simulink model "AR4FullPositionControl"  (R2026a)
settings: Solver=FixedStepAuto  StopTime=inf  FixedStep=3e-5
PreLoadFcn:
  | load('last_pos.mat');
StopFcn:
  | save('last_pos.mat', 'posJ6', 'posJ5', 'posJ4', 'posJ3', 'posJ2', 'posJ1', 'lastX', 'lastY', 'lastZ');
undefined symbols (not defined in the file): targetColor, targetGo, targetX, targetY, targetZ
libraries: arduinolib x31
(part 1 of 3)
settings Model: SILPILModeSetting=veronly  ExtModeTrigDuration=2  TunableVars=px  TunableVarsStorageClass=ExportedGlobal  Creator=abdnuris  LastModifiedBy=abdnuris
settings HardwareCC: ProdLargestAtomicInteger=Long  ProdLargestAtomicFloat=Double  ProdHWDeviceType=ARM Compatible->ARM Cortex
settings RTWCC: SystemTargetFile=ert.tlc  HardwareBoard=Teensy 4.1 (Arduino Compatible)  TLCOptions=-aInlineSetEventsForThisBaseRateFcn=TLC_FALSE -aSuppressMultiTaskScheduler=TLC_FALSE -aRateBasedStepFcn=1  Toolchain=Arduino ARM M7  Description=Embedded Coder
settings ERTTargetCC: ExtModeTransport=3.0  ExtModeAutomaticAllocSize=off  ExtModeStaticAllocSize=65536.0  SupportContinuousTime=on  SupportVariableSizeSignals=on

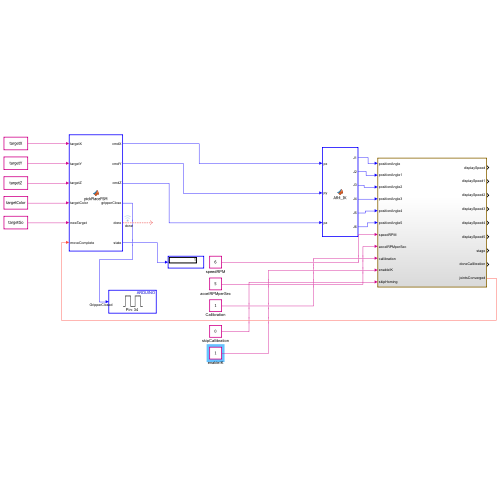
[thumbnail: Simulink's stored preview of the top-level diagram]
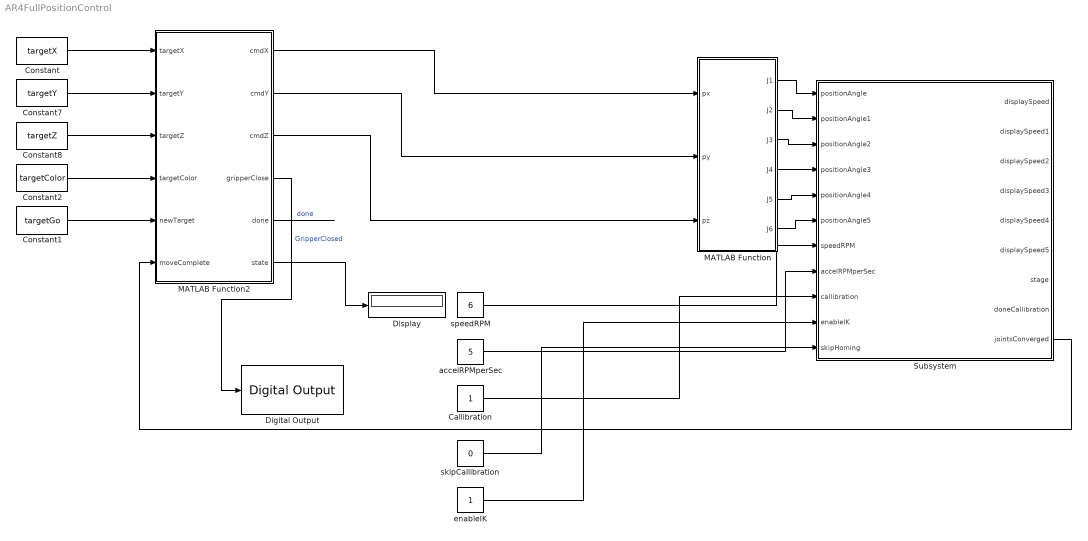
== system AR4FullPositionControl ==
  Callibration : Constant
  Constant : Constant  Value=targetX
  Constant1 : Constant  Value=targetGo
  Constant2 : Constant  Value=targetColor
  Constant7 : Constant  Value=targetY
  Constant8 : Constant  Value=targetZ
  Digital Output : arduinolib/Digital Output  pinNumber=34  Direction=output  blockPlatform=arduino
  Display : Display
  MATLAB Function : MATLAB Function  TreatAsAtomicUnit=on  SystemSampleTime=0.0075
  MATLAB Function2 : MATLAB Function  TreatAsAtomicUnit=on  SystemSampleTime=0.03
  Subsystem : Subsystem
  accelRPMperSec : Constant  Value=5
  enableIK : Constant
  skipCallibration : Constant  Value=0
  speedRPM : Constant  Value=6
  wires:
  MATLAB Function/2(J2) -> Subsystem/2(positionAngle1)
  MATLAB Function/3(J3) -> Subsystem/3(positionAngle2)
  MATLAB Function/4(J4) -> Subsystem/4(positionAngle3)
  MATLAB Function/5(J5) -> Subsystem/5(positionAngle4)
  MATLAB Function/6(J6) -> Subsystem/6(positionAngle5)
  MATLAB Function/1(J1) -> Subsystem/1(positionAngle)
  speedRPM/1 -> Subsystem/7(speedRPM)
  accelRPMperSec/1 -> Subsystem/8(accelRPMperSec)
  Callibration/1 -> Subsystem/9(callibration)
  enableIK/1 -> Subsystem/10(enableIK)
  MATLAB Function2/4(gripperClose) -> Digital Output/1  "GripperClosed"
  skipCallibration/1 -> Subsystem/11(skipHoming)
  Constant7/1 -> MATLAB Function2/2(targetY)
  Constant/1 -> MATLAB Function2/1(targetX)
  Constant8/1 -> MATLAB Function2/3(targetZ)
  Constant1/1 -> MATLAB Function2/5(newTarget)
  MATLAB Function2/5(done) -> ?  "done"
  Subsystem/9(jointsConverged) -> MATLAB Function2/6(moveComplete)
  MATLAB Function2/6(state) -> Display/1
  MATLAB Function2/1(cmdX) -> MATLAB Function/1(px)
  MATLAB Function2/3(cmdZ) -> MATLAB Function/3(pz)
  MATLAB Function2/2(cmdY) -> MATLAB Function/2(py)
  Constant2/1 -> MATLAB Function2/4(targetColor)

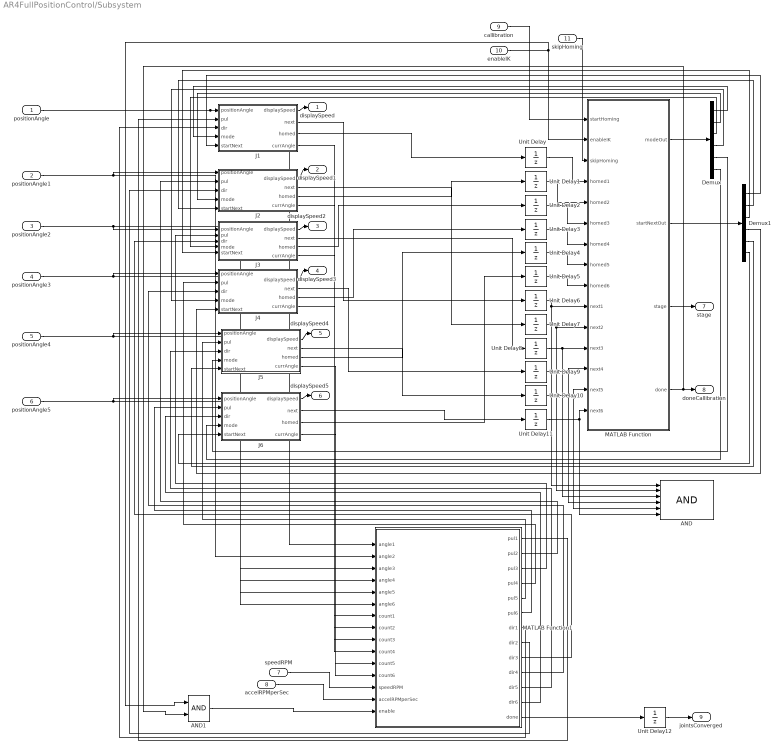
== system AR4FullPositionControl/Subsystem ==
  positionAngle : Inport
  positionAngle1 : Inport  Port=2
  positionAngle2 : Inport  Port=3
  positionAngle3 : Inport  Port=4
  positionAngle4 : Inport  Port=5
  positionAngle5 : Inport  Port=6
  speedRPM : Inport  Port=7
  accelRPMperSec : Inport  Port=8
  callibration : Inport  Port=9
  enableIK : Inport  Port=10
  skipHoming : Inport  Port=11
  AND : Logic  Inputs=6  IconShape=distinctive  AllPortsSameDT=off  OutDataTypeStr=boolean
  AND1 : Logic  IconShape=distinctive  AllPortsSameDT=off  OutDataTypeStr=boolean
  Demux : Demux  Outputs=6
  Demux1 : Demux  Outputs=6
  J1 : Subsystem
  J2 : Subsystem
  J3 : Subsystem
  J4 : Subsystem
  J5 : Subsystem
  J6 : Subsystem
  MATLAB Function : MATLAB Function  TreatAsAtomicUnit=on  SystemSampleTime=0.0075
  MATLAB Function1 : MATLAB Function  TreatAsAtomicUnit=on  SystemSampleTime=3e-5
  Unit Delay{,1..11} (12 alike) : UnitDelay  SampleTime=-1
  Unit Delay12 : UnitDelay  InitialCondition=false  SampleTime=-1
  displaySpeed : Outport
  displaySpeed1 : Outport  Port=2
  displaySpeed2 : Outport  Port=3
  displaySpeed3 : Outport  Port=4
  displaySpeed4 : Outport  Port=5
  displaySpeed5 : Outport  Port=6
  stage : Outport  Port=7
  doneCallibration : Outport  Port=8
  jointsConverged : Outport  Port=9
  wires:
  positionAngle4/1 -> MATLAB Function1/5(angle5), J5/1(positionAngle)
  MATLAB Function1/6(pul6) -> J6/2(pul)
  J2/2(next) -> Unit Delay7/1
  J6/1(displaySpeed) -> displaySpeed5/1
  positionAngle5/1 -> MATLAB Function1/6(angle6), J6/1(positionAngle)
  J3/2(next) -> Unit Delay8/1
  positionAngle2/1 -> MATLAB Function1/3(angle3), J3/1(positionAngle)
  J4/2(next) -> Unit Delay9/1
  positionAngle1/1 -> MATLAB Function1/2(angle2), J2/1(positionAngle)
  positionAngle/1 -> MATLAB Function1/1(angle1), J1/1(positionAngle)
  positionAngle3/1 -> MATLAB Function1/4(angle4), J4/1(positionAngle)
  J2/1(displaySpeed) -> displaySpeed1/1
  J4/1(displaySpeed) -> displaySpeed3/1
  J5/1(displaySpeed) -> displaySpeed4/1
  J3/1(displaySpeed) -> displaySpeed2/1
  J5/2(next) -> Unit Delay10/1
  J1/1(displaySpeed) -> displaySpeed/1
  J6/2(next) -> Unit Delay11/1
  MATLAB Function1/12(dir6) -> J6/3(dir)
  J1/3(homed) -> Unit Delay/1
  J2/3(homed) -> Unit Delay1/1
  J3/3(homed) -> Unit Delay2/1
  J4/3(homed) -> Unit Delay3/1
  J5/3(homed) -> Unit Delay4/1
  J6/3(homed) -> Unit Delay5/1
  callibration/1 -> MATLAB Function/1(startHoming)
  MATLAB Function/1(modeOut) -> Demux/1
  Demux/1 -> J1/4(mode)
  Demux/2 -> J2/4(mode)
  Demux/3 -> J3/4(mode)
  Demux/4 -> J4/4(mode)
  Demux/5 -> J5/4(mode)
  Demux/6 -> J6/4(mode)
  MATLAB Function/2(startNextOut) -> Demux1/1
  Demux1/1 -> J1/5(startNext)
  Demux1/2 -> J2/5(startNext)
  Demux1/3 -> J3/5(startNext)
  Demux1/4 -> J4/5(startNext)
  Demux1/5 -> J5/5(startNext)
  Demux1/6 -> J6/5(startNext)
  enableIK/1 -> MATLAB Function/2(enableIK), AND1/1
  MATLAB Function/3(stage) -> stage/1
  MATLAB Function/4(done) -> AND1/2, doneCallibration/1
  Unit Delay/1 -> MATLAB Function/4(homed1)
  Unit Delay1/1 -> MATLAB Function/5(homed2)
  Unit Delay2/1 -> MATLAB Function/6(homed3)
  Unit Delay3/1 -> MATLAB Function/7(homed4)
  Unit Delay4/1 -> MATLAB Function/8(homed5)
  Unit Delay5/1 -> MATLAB Function/9(homed6)
  Unit Delay6/1 -> AND/1, MATLAB Function/10(next1)
  Unit Delay7/1 -> AND/2, MATLAB Function/11(next2)
  Unit Delay8/1 -> AND/3, MATLAB Function/12(next3)
  Unit Delay9/1 -> AND/4, MATLAB Function/13(next4)
  Unit Delay10/1 -> AND/5, MATLAB Function/14(next5)
  Unit Delay11/1 -> AND/6, MATLAB Function/15(next6)
  J1/2(next) -> Unit Delay6/1
  J1/4(currAngle) -> MATLAB Function1/7(count1)
  J2/4(currAngle) -> MATLAB Function1/8(count2)
  J3/4(currAngle) -> MATLAB Function1/9(count3)
  J4/4(currAngle) -> MATLAB Function1/10(count4)
  J5/4(currAngle) -> MATLAB Function1/11(count5)
  J6/4(currAngle) -> MATLAB Function1/12(count6)
  speedRPM/1 -> MATLAB Function1/13(speedRPM)
  accelRPMperSec/1 -> MATLAB Function1/14(accelRPMperSec)
  MATLAB Function1/1(pul1) -> J1/2(pul)
  MATLAB Function1/2(pul2) -> J2/2(pul)
  MATLAB Function1/3(pul3) -> J3/2(pul)
  MATLAB Function1/4(pul4) -> J4/2(pul)
  MATLAB Function1/5(pul5) -> J5/2(pul)
  MATLAB Function1/10(dir4) -> J4/3(dir)
  MATLAB Function1/8(dir2) -> J2/3(dir)
  MATLAB Function1/7(dir1) -> J1/3(dir)
  MATLAB Function1/11(dir5) -> J5/3(dir)
  MATLAB Function1/9(dir3) -> J3/3(dir)
  skipHoming/1 -> MATLAB Function/3(skipHoming)
  Unit Delay12/1 -> jointsConverged/1
  MATLAB Function1/13(done) -> Unit Delay12/1
  AND1/1 -> MATLAB Function1/15(enable)

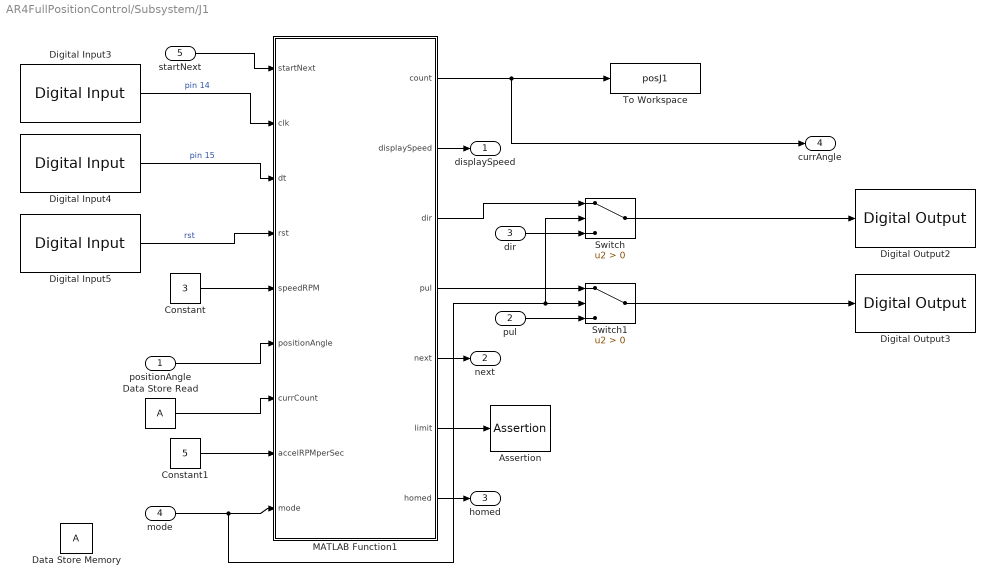
== system AR4FullPositionControl/Subsystem/J1 ==
  positionAngle : Inport
  pul : Inport  Port=2
  dir : Inport  Port=3
  mode : Inport  Port=4
  startNext : Inport  Port=5
  Assertion : Assertion  AssertionFailFcn="error(\"Limit J1\")"
  Constant : Constant  Value=3
  Constant1 : Constant  Value=5
  Data Store Memory : DataStoreMemory  WriteAfterWriteMsg=warning  InitialValue=posJ1  ShowAdditionalParam=off
  Data Store Read : DataStoreRead  IndexOptions=Index vector (dialog)  Indices=1  OutputSizes=1
  Digital Input3 : arduinolib/Digital Input  pinNumber=14  mode=Default  Direction=input  SampleTime=-1  blockPlatform=arduino
  Digital Input4 : arduinolib/Digital Input  pinNumber=15  mode=Default  Direction=input  SampleTime=-1  blockPlatform=arduino
  Digital Input5 : arduinolib/Digital Input  pinNumber=26  mode=Default  Direction=input  SampleTime=0.0015  blockPlatform=arduino
  Digital Output2 : arduinolib/Digital Output  pinNumber=1  Direction=output  blockPlatform=arduino
  Digital Output3 : arduinolib/Digital Output  pinNumber=0  Direction=output  blockPlatform=arduino
  MATLAB Function1 : MATLAB Function  TreatAsAtomicUnit=on  SystemSampleTime=3e-5
  Switch : Switch  Criteria=u2 > Threshold  SaturateOnIntegerOverflow=off  InputSameDT=off
  Switch1 : Switch  Criteria=u2 > Threshold  SaturateOnIntegerOverflow=off  InputSameDT=off
  To Workspace : ToWorkspace  VariableName=posJ1  SampleTime=0.0075
      settings: MaxDataPoints=1  Decimation=2
  displaySpeed : Outport
  next : Outport  Port=2
  homed : Outport  Port=3
  currAngle : Outport  Port=4
  wires:
  MATLAB Function1/6(limit) -> Assertion/1
  Digital Input4/1 -> MATLAB Function1/3(dt)  "pin 15"
  Data Store Read/1 -> MATLAB Function1/7(currCount)
  startNext/1 -> MATLAB Function1/1(startNext)
  Digital Input3/1 -> MATLAB Function1/2(clk)  "pin 14"
  Digital Input5/1 -> MATLAB Function1/4(rst)  "rst"
  positionAngle/1 -> MATLAB Function1/6(positionAngle)
  MATLAB Function1/2(displaySpeed) -> displaySpeed/1
  MATLAB Function1/5(next) -> next/1
  MATLAB Function1/7(homed) -> homed/1
  MATLAB Function1/1(count) -> currAngle/1, To Workspace/1
  Switch1/1 -> Digital Output3/1
  MATLAB Function1/3(dir) -> Switch/1
  mode/1 -> Switch1/2, Switch/2, MATLAB Function1/9(mode)
  MATLAB Function1/4(pul) -> Switch1/1
  dir/1 -> Switch/3
  pul/1 -> Switch1/3
  Switch/1 -> Digital Output2/1
  Constant/1 -> MATLAB Function1/5(speedRPM)
  Constant1/1 -> MATLAB Function1/8(accelRPMperSec)

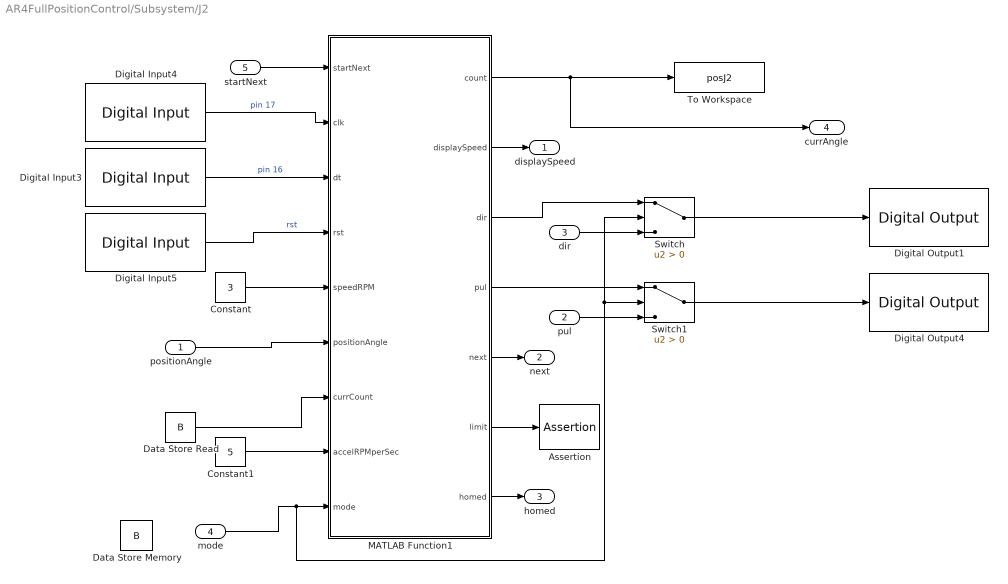
== system AR4FullPositionControl/Subsystem/J2 ==
  positionAngle : Inport
  pul : Inport  Port=2
  dir : Inport  Port=3
  mode : Inport  Port=4
  startNext : Inport  Port=5
  Assertion : Assertion  AssertionFailFcn="error(\"Limit J2\")"
  Constant : Constant  Value=3
  Constant1 : Constant  Value=5
  Data Store Memory : DataStoreMemory  DataStoreName=B  WriteAfterWriteMsg=warning  InitialValue=posJ2  ShowAdditionalParam=off
  Data Store Read : DataStoreRead  DataStoreName=B  IndexOptions=Index vector (dialog)  Indices=1  OutputSizes=1
  Digital Input3 : arduinolib/Digital Input  pinNumber=16  mode=Default  Direction=input  SampleTime=-1  blockPlatform=arduino
  Digital Input4 : arduinolib/Digital Input  pinNumber=17  mode=Default  Direction=input  SampleTime=-1  blockPlatform=arduino
  Digital Input5 : arduinolib/Digital Input  pinNumber=27  mode=Default  Direction=input  SampleTime=0.0015  blockPlatform=arduino
  Digital Output1 : arduinolib/Digital Output  pinNumber=3  Direction=output  blockPlatform=arduino
  Digital Output4 : arduinolib/Digital Output  pinNumber=2  Direction=output  blockPlatform=arduino
  MATLAB Function1 : MATLAB Function  TreatAsAtomicUnit=on
  Switch : Switch  Criteria=u2 > Threshold  SaturateOnIntegerOverflow=off  InputSameDT=off
  Switch1 : Switch  Criteria=u2 > Threshold  SaturateOnIntegerOverflow=off  InputSameDT=off
  To Workspace : ToWorkspace  VariableName=posJ2  SampleTime=0.0075
      settings: MaxDataPoints=1  Decimation=2
  displaySpeed : Outport
  next : Outport  Port=2
  homed : Outport  Port=3
  currAngle : Outport  Port=4
  wires:
  Digital Input4/1 -> MATLAB Function1/2(clk)  "pin 17"
  Digital Input5/1 -> MATLAB Function1/4(rst)  "rst"
  Digital Input3/1 -> MATLAB Function1/3(dt)  "pin 16"
  Data Store Read/1 -> MATLAB Function1/7(currCount)
  MATLAB Function1/6(limit) -> Assertion/1
  MATLAB Function1/5(next) -> next/1
  MATLAB Function1/2(displaySpeed) -> displaySpeed/1
  positionAngle/1 -> MATLAB Function1/6(positionAngle)
  MATLAB Function1/7(homed) -> homed/1
  startNext/1 -> MATLAB Function1/1(startNext)
  MATLAB Function1/1(count) -> currAngle/1, To Workspace/1
  MATLAB Function1/4(pul) -> Switch1/1
  MATLAB Function1/3(dir) -> Switch/1
  Switch1/1 -> Digital Output4/1
  Switch/1 -> Digital Output1/1
  mode/1 -> Switch/2, Switch1/2, MATLAB Function1/9(mode)
  pul/1 -> Switch1/3
  dir/1 -> Switch/3
  Constant/1 -> MATLAB Function1/5(speedRPM)
  Constant1/1 -> MATLAB Function1/8(accelRPMperSec)

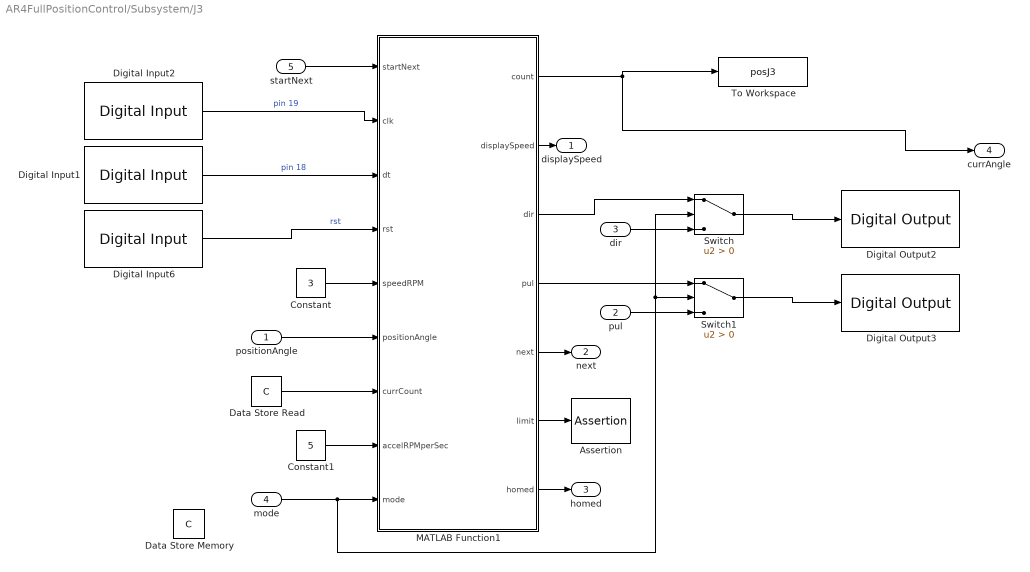
== system AR4FullPositionControl/Subsystem/J3 ==
  positionAngle : Inport
  pul : Inport  Port=2
  dir : Inport  Port=3
  mode : Inport  Port=4
  startNext : Inport  Port=5
  Assertion : Assertion  AssertionFailFcn="error(\"Limit J3\")"
  Constant : Constant  Value=3
  Constant1 : Constant  Value=5
  Data Store Memory : DataStoreMemory  DataStoreName=C  WriteAfterWriteMsg=warning  InitialValue=posJ3  ShowAdditionalParam=off
  Data Store Read : DataStoreRead  DataStoreName=C  IndexOptions=Index vector (dialog)  Indices=1  OutputSizes=1
  Digital Input1 : arduinolib/Digital Input  pinNumber=18  mode=Default  Direction=input  SampleTime=-1  blockPlatform=arduino
  Digital Input2 : arduinolib/Digital Input  pinNumber=19  mode=Default  Direction=input  SampleTime=-1  blockPlatform=arduino
  Digital Input6 : arduinolib/Digital Input  pinNumber=28  mode=Default  Direction=input  SampleTime=0.0015  blockPlatform=arduino
  Digital Output2 : arduinolib/Digital Output  pinNumber=5  Direction=output  blockPlatform=arduino
  Digital Output3 : arduinolib/Digital Output  pinNumber=4  Direction=output  blockPlatform=arduino
  MATLAB Function1 : MATLAB Function  TreatAsAtomicUnit=on
  Switch : Switch  Criteria=u2 > Threshold  SaturateOnIntegerOverflow=off  InputSameDT=off
  Switch1 : Switch  Criteria=u2 > Threshold  SaturateOnIntegerOverflow=off  InputSameDT=off
  To Workspace : ToWorkspace  VariableName=posJ3  SampleTime=0.0075
      settings: MaxDataPoints=1  Decimation=2
  displaySpeed : Outport
  next : Outport  Port=2
  homed : Outport  Port=3
  currAngle : Outport  Port=4
  wires:
  Digital Input1/1 -> MATLAB Function1/3(dt)  "pin 18"
  Digital Input2/1 -> MATLAB Function1/2(clk)  "pin 19"
  Digital Input6/1 -> MATLAB Function1/4(rst)  "rst"
  Data Store Read/1 -> MATLAB Function1/7(currCount)
  MATLAB Function1/6(limit) -> Assertion/1
  positionAngle/1 -> MATLAB Function1/6(positionAngle)
  MATLAB Function1/2(displaySpeed) -> displaySpeed/1
  MATLAB Function1/5(next) -> next/1
  MATLAB Function1/7(homed) -> homed/1
  startNext/1 -> MATLAB Function1/1(startNext)
  MATLAB Function1/1(count) -> currAngle/1, To Workspace/1
  Switch/1 -> Digital Output2/1
  Switch1/1 -> Digital Output3/1
  MATLAB Function1/3(dir) -> Switch/1
  MATLAB Function1/4(pul) -> Switch1/1
  mode/1 -> Switch/2, Switch1/2, MATLAB Function1/9(mode)
  dir/1 -> Switch/3
  pul/1 -> Switch1/3
  Constant/1 -> MATLAB Function1/5(speedRPM)
  Constant1/1 -> MATLAB Function1/8(accelRPMperSec)

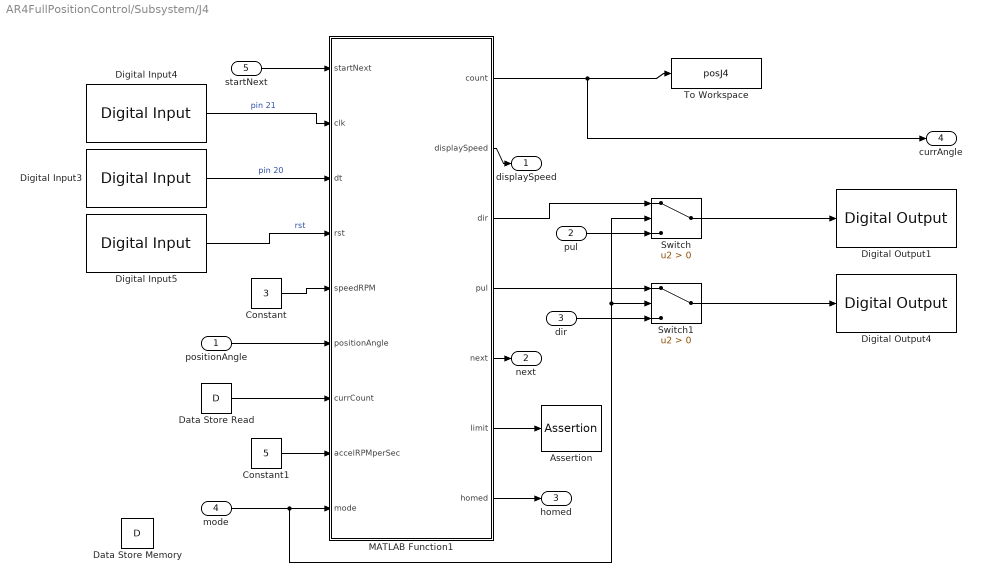
== system AR4FullPositionControl/Subsystem/J4 ==
  positionAngle : Inport
  pul : Inport  Port=2
  dir : Inport  Port=3
  mode : Inport  Port=4
  startNext : Inport  Port=5
  Assertion : Assertion  AssertionFailFcn="error(\"Limit J4\")"
  Constant : Constant  Value=3
  Constant1 : Constant  Value=5
  Data Store Memory : DataStoreMemory  DataStoreName=D  WriteAfterWriteMsg=warning  InitialValue=posJ4  ShowAdditionalParam=off
  Data Store Read : DataStoreRead  DataStoreName=D  IndexOptions=Index vector (dialog)  Indices=1  OutputSizes=1
  Digital Input3 : arduinolib/Digital Input  pinNumber=20  mode=Default  Direction=input  SampleTime=-1  blockPlatform=arduino
  Digital Input4 : arduinolib/Digital Input  pinNumber=21  mode=Default  Direction=input  SampleTime=-1  blockPlatform=arduino
  Digital Input5 : arduinolib/Digital Input  pinNumber=29  mode=Default  Direction=input  SampleTime=0.0015  blockPlatform=arduino
  Digital Output1 : arduinolib/Digital Output  pinNumber=7  Direction=output  blockPlatform=arduino
  Digital Output4 : arduinolib/Digital Output  pinNumber=6  Direction=output  blockPlatform=arduino
  MATLAB Function1 : MATLAB Function  TreatAsAtomicUnit=on
  Switch : Switch  Criteria=u2 > Threshold  SaturateOnIntegerOverflow=off  InputSameDT=off
  Switch1 : Switch  Criteria=u2 > Threshold  SaturateOnIntegerOverflow=off  InputSameDT=off
  To Workspace : ToWorkspace  VariableName=posJ4  SampleTime=0.0075
      settings: MaxDataPoints=1  Decimation=2
  displaySpeed : Outport
  next : Outport  Port=2
  homed : Outport  Port=3
  currAngle : Outport  Port=4
  wires:
  Digital Input5/1 -> MATLAB Function1/4(rst)  "rst"
  Digital Input3/1 -> MATLAB Function1/3(dt)  "pin 20"
  Data Store Read/1 -> MATLAB Function1/7(currCount)
  MATLAB Function1/6(limit) -> Assertion/1
  Digital Input4/1 -> MATLAB Function1/2(clk)  "pin 21"
  MATLAB Function1/2(displaySpeed) -> displaySpeed/1
  MATLAB Function1/5(next) -> next/1
  positionAngle/1 -> MATLAB Function1/6(positionAngle)
  MATLAB Function1/7(homed) -> homed/1
  startNext/1 -> MATLAB Function1/1(startNext)
  MATLAB Function1/1(count) -> currAngle/1, To Workspace/1
  dir/1 -> Switch1/3
  Switch/1 -> Digital Output1/1
  MATLAB Function1/3(dir) -> Switch/1
  pul/1 -> Switch/3
  MATLAB Function1/4(pul) -> Switch1/1
  Switch1/1 -> Digital Output4/1
  mode/1 -> Switch/2, Switch1/2, MATLAB Function1/9(mode)
  Constant/1 -> MATLAB Function1/5(speedRPM)
  Constant1/1 -> MATLAB Function1/8(accelRPMperSec)

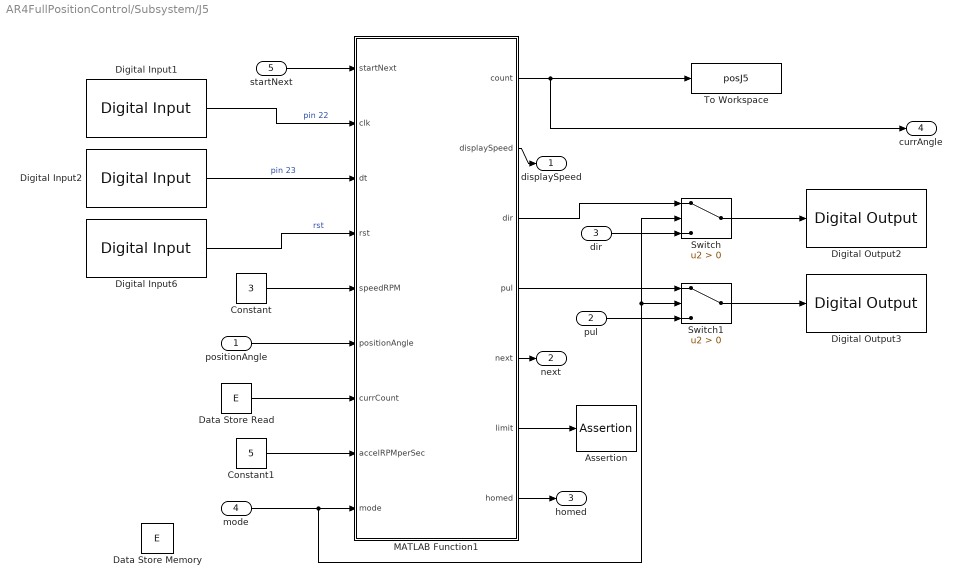
== system AR4FullPositionControl/Subsystem/J5 ==
  positionAngle : Inport
  pul : Inport  Port=2
  dir : Inport  Port=3
  mode : Inport  Port=4
  startNext : Inport  Port=5
  Assertion : Assertion  AssertionFailFcn="error(\"Limit J5\")"
  Constant : Constant  Value=3
  Constant1 : Constant  Value=5
  Data Store Memory : DataStoreMemory  DataStoreName=E  WriteAfterWriteMsg=warning  InitialValue=posJ5  ShowAdditionalParam=off
  Data Store Read : DataStoreRead  DataStoreName=E  IndexOptions=Index vector (dialog)  Indices=1  OutputSizes=1
  Digital Input1 : arduinolib/Digital Input  pinNumber=22  mode=Default  Direction=input  SampleTime=-1  blockPlatform=arduino
  Digital Input2 : arduinolib/Digital Input  pinNumber=23  mode=Default  Direction=input  SampleTime=-1  blockPlatform=arduino
  Digital Input6 : arduinolib/Digital Input  pinNumber=30  mode=Default  Direction=input  SampleTime=0.006  blockPlatform=arduino
  Digital Output2 : arduinolib/Digital Output  pinNumber=9  Direction=output  blockPlatform=arduino
  Digital Output3 : arduinolib/Digital Output  pinNumber=8  Direction=output  blockPlatform=arduino
  MATLAB Function1 : MATLAB Function  TreatAsAtomicUnit=on
  Switch : Switch  Criteria=u2 > Threshold  SaturateOnIntegerOverflow=off  InputSameDT=off
  Switch1 : Switch  Criteria=u2 > Threshold  SaturateOnIntegerOverflow=off  InputSameDT=off
  To Workspace : ToWorkspace  VariableName=posJ5  SampleTime=0.0075
      settings: MaxDataPoints=1  Decimation=2
  displaySpeed : Outport
  next : Outport  Port=2
  homed : Outport  Port=3
  currAngle : Outport  Port=4
  wires:
  MATLAB Function1/5(next) -> next/1
  Digital Input2/1 -> MATLAB Function1/3(dt)  "pin 23"
  Data Store Read/1 -> MATLAB Function1/7(currCount)
  Digital Input6/1 -> MATLAB Function1/4(rst)  "rst"
  MATLAB Function1/6(limit) -> Assertion/1
  Digital Input1/1 -> MATLAB Function1/2(clk)  "pin 22"
  positionAngle/1 -> MATLAB Function1/6(positionAngle)
  MATLAB Function1/2(displaySpeed) -> displaySpeed/1
  MATLAB Function1/7(homed) -> homed/1
  startNext/1 -> MATLAB Function1/1(startNext)
  MATLAB Function1/1(count) -> currAngle/1, To Workspace/1
  Switch1/1 -> Digital Output3/1
  MATLAB Function1/3(dir) -> Switch/1
  Switch/1 -> Digital Output2/1
  MATLAB Function1/4(pul) -> Switch1/1
  mode/1 -> Switch/2, Switch1/2, MATLAB Function1/9(mode)
  pul/1 -> Switch1/3
  dir/1 -> Switch/3
  Constant/1 -> MATLAB Function1/5(speedRPM)
  Constant1/1 -> MATLAB Function1/8(accelRPMperSec)

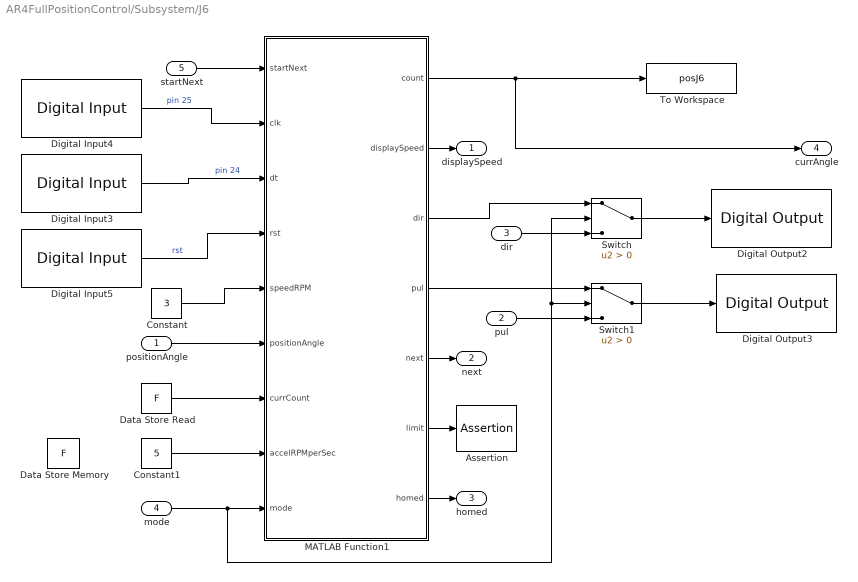
== system AR4FullPositionControl/Subsystem/J6 ==
  positionAngle : Inport
  pul : Inport  Port=2
  dir : Inport  Port=3
  mode : Inport  Port=4
  startNext : Inport  Port=5
  Assertion : Assertion  AssertionFailFcn="error(\"Limit J6\")"
  Constant : Constant  Value=3
  Constant1 : Constant  Value=5
  Data Store Memory : DataStoreMemory  DataStoreName=F  WriteAfterWriteMsg=warning  InitialValue=posJ6  ShowAdditionalParam=off
  Data Store Read : DataStoreRead  DataStoreName=F  IndexOptions=Index vector (dialog)  Indices=1  OutputSizes=1
  Digital Input3 : arduinolib/Digital Input  pinNumber=24  mode=Default  Direction=input  SampleTime=-1  blockPlatform=arduino
  Digital Input4 : arduinolib/Digital Input  pinNumber=25  mode=Default  Direction=input  SampleTime=-1  blockPlatform=arduino
  Digital Input5 : arduinolib/Digital Input  pinNumber=31  mode=Default  Direction=input  SampleTime=0.003  blockPlatform=arduino
  Digital Output2 : arduinolib/Digital Output  pinNumber=11  Direction=output  blockPlatform=arduino
  Digital Output3 : arduinolib/Digital Output  pinNumber=10  Direction=output  blockPlatform=arduino
  MATLAB Function1 : MATLAB Function  TreatAsAtomicUnit=on
  Switch : Switch  Criteria=u2 > Threshold  SaturateOnIntegerOverflow=off  InputSameDT=off
  Switch1 : Switch  Criteria=u2 > Threshold  SaturateOnIntegerOverflow=off  InputSameDT=off
  To Workspace : ToWorkspace  VariableName=posJ6  SampleTime=0.0075
      settings: MaxDataPoints=1  Decimation=2
  displaySpeed : Outport
  next : Outport  Port=2
  homed : Outport  Port=3
  currAngle : Outport  Port=4
  wires:
  Digital Input5/1 -> MATLAB Function1/4(rst)  "rst"
  MATLAB Function1/6(limit) -> Assertion/1
  Digital Input4/1 -> MATLAB Function1/2(clk)  "pin 25"
  MATLAB Function1/2(displaySpeed) -> displaySpeed/1
  Digital Input3/1 -> MATLAB Function1/3(dt)  "pin 24"
  Data Store Read/1 -> MATLAB Function1/7(currCount)
  MATLAB Function1/5(next) -> next/1
  mode/1 -> Switch/2, Switch1/2, MATLAB Function1/9(mode)
  MATLAB Function1/7(homed) -> homed/1
  startNext/1 -> MATLAB Function1/1(startNext)
  MATLAB Function1/1(count) -> currAngle/1, To Workspace/1
  Switch/1 -> Digital Output2/1
  MATLAB Function1/3(dir) -> Switch/1
  pul/1 -> Switch1/3
  MATLAB Function1/4(pul) -> Switch1/1
  Switch1/1 -> Digital Output3/1
  positionAngle/1 -> MATLAB Function1/6(positionAngle)
  dir/1 -> Switch/3
  Constant/1 -> MATLAB Function1/5(speedRPM)
  Constant1/1 -> MATLAB Function1/8(accelRPMperSec)

== matlab function AR4FullPositionControl/Subsystem/J4/MATLAB Function1 ==
  data: startNext input; clk input; count output; dt input; rst input; displaySpeed output; dir output; pul output; next output; speedRPM input; positionAngle input; currCount input; accelRPMperSec input; limit output; mode input; homed output
function [count, displaySpeed, dir, pul, next, limit, homed] = J4(startNext, clk, dt, rst, speedRPM, positionAngle, currCount, accelRPMperSec, mode)
% J4 - Joint 4 position/speed controller with S-curve acceleration + HOMING
%
% AR4-MK3 robot. ZERO_COUNT template (rotational, dual-limit).
% Switch at the most-negative-angle end = count 0.
% 0 deg corresponds to count = ZERO_COUNT.
%
% MODE (single input):
%   mode = 0  ->  POSITION  : normal operation, drive to positionAngle input
%   mode = 1  ->  INITIALIZE: drive to HOME_TARGET, ignore positionAngle
%   mode = 2  ->  HOMING    : drive toward limit switch, zero count on contact
%
%   >>> J4: ZERO_COUNT=22238  maxCount=42860

    persistent currentCount lastClkState lastCount spTimer smoothedSpeed ...
               currentRPM distTraveled totalMoveFrozen lastTarget pulseAccum ...
               homedFlag lastMode;

    % -------------------------------------------------------------------------
    % CONSTANTS
    % -------------------------------------------------------------------------
    Ts           = 3e-5;
    PPR          = 1000;
    CPR          = PPR * 4;
    maxCount     = 42860;          % <<< J4
    LIMIT_BUFFER = 50;
    TUNE_C2R     = 0.8;            % <<< J4
    TOTAL_DEG    = 179 + 165;      % <<< J4 span = 344
    COUNTS_PER_REV = maxCount / TOTAL_DEG * 360;
    GEAR_RATIO     = COUNTS_PER_REV / CPR;
    C2R            = (GEAR_RATIO * CPR) / 60 * TUNE_C2R;

    speedUpdateInterval = 0.2;
    ALPHA               = 0.3;
    MIN_RPM             = 0.5;
    STOP_COUNTS         = 1;

    HOME_RPM    = 5;               % <<< tune: homing speed (RPM)
    HOME_TARGET = 0;               % <<< angle commanded in mode=1 (deg)

    ZERO_COUNT   = 22238;          % <<< J4 count at 0 deg
    countsPerDeg = maxCount / TOTAL_DEG;

    % -------------------------------------------------------------------------
    % INITIALISATION (first call only)
    % -------------------------------------------------------------------------
    if isempty(currentCount)
        currentCount    = currCount;
        lastCount       = currCount;
        lastClkState    = clk;
        spTimer         = 0;
        smoothedSpeed   = 0;
        currentRPM      = MIN_RPM;
        distTraveled    = 0;
        totalMoveFrozen = 0;
        lastTarget      = -1;
        pulseAccum      = 0;
        homedFlag       = false;
        lastMode        = 0;
    end

    limit = false;
    homed = homedFlag;
    dir   = 0;
    pul   = 0;
    next  = false;

    % -------------------------------------------------------------------------
    % 1. ENCODER COUNTING
    % -------------------------------------------------------------------------
    if clk ~= lastClkState && clk == 1
        if dt ~= clk
            currentCount = currentCount + 1;
        else
            currentCount = currentCount - 1;
        end
    end

    % Reset S-curve state on any mode change
    if mode ~= lastMode
        distTraveled    = 0;
        totalMoveFrozen = 0;
        pulseAccum      = 0;
        lastTarget      = -1;
        currentRPM      = MIN_RPM;
        spTimer         = 0;
        smoothedSpeed   = 0;
    end
    lastMode = mode;

    % =========================================================================
    % MODE 2: HOMING
    % =========================================================================
    if mode == 2
        if rst == 1
            currentCount = 0;
            homedFlag    = true;
        end
        homed = homedFlag;

        if homedFlag
            currentCount = 0;
            pul          = 0;
            next         = true;
        elseif startNext
            dir        = 0;        % toward switch = decreasing count
            pulseAccum = pulseAccum + HOME_RPM * C2R * Ts;
            if pulseAccum >= 1.0
                pul        = 1;
                pulseAccum = pulseAccum - 1.0;
            end
        end

        count        = currentCount;
        displaySpeed = HOME_RPM;
        lastClkState = clk;
        return;
    end
    % =========================================================================

    % -------------------------------------------------------------------------
    % 2. SPEED DISPLAY
    % -------------------------------------------------------------------------
    spTimer = spTimer + Ts;
    if spTimer >= speedUpdateInterval
        smoothedSpeed = ALPHA * currentRPM + (1 - ALPHA) * smoothedSpeed;
        spTimer       = 0;
    end

    % -------------------------------------------------------------------------
    % 3. TARGET FROM ANGLE  (ZERO_COUNT anchor)
    %    mode 1: command = HOME_TARGET ; mode 0: command = positionAngle
    % -------------------------------------------------------------------------
    if mode == 1
        cmdAngle = HOME_TARGET;
    else
        cmdAngle = positionAngle;
    end

    targetCount = round(ZERO_COUNT + cmdAngle * countsPerDeg);
    targetCount = max(LIMIT_BUFFER, min(maxCount - LIMIT_BUFFER, targetCount));

    % -------------------------------------------------------------------------
    % 4. DIRECTION
    % -------------------------------------------------------------------------
    countError = targetCount - currentCount;
    absError   = abs(countError);
    if countError >= 0
        dir = 1;
    else
        dir = 0;
    end

    % -------------------------------------------------------------------------
    % 5. FREEZE totalMove ON NEW TARGET
    % -------------------------------------------------------------------------
    if targetCount ~= lastTarget
        totalMoveFrozen = absError;
        distTraveled    = 0;
        pulseAccum      = 0;
        lastTarget      = targetCount;
    end

    % -------------------------------------------------------------------------
    % 6. S-CURVE SPEED PROFILE
    % -------------------------------------------------------------------------
    accel = max(accelRPMperSec, 0.1);
    fullRampCounts = 0.5 * (MIN_RPM + speedRPM) * C2R * (speedRPM - MIN_RPM) / accel;

    if totalMoveFrozen > 0 && 2 * fullRampCounts >= totalMoveFrozen
        peakRPM    = sqrt(max(MIN_RPM^2 + totalMoveFrozen * accel / C2R, MIN_RPM^2));
        peakRPM    = max(MIN_RPM, min(speedRPM, peakRPM));
        rampCounts = 0.5 * (MIN_RPM + peakRPM) * C2R * (peakRPM - MIN_RPM) / accel;
        rampCounts = max(1, rampCounts);
    else
        peakRPM    = speedRPM;
        rampCounts = max(1, fullRampCounts);
    end

    if totalMoveFrozen <= 0
        targetRPM = MIN_RPM;
    elseif absError <= rampCounts
        x         = max(0.0, min(1.0, absError / rampCounts));
        targetRPM = MIN_RPM + (peakRPM - MIN_RPM) * 0.5 * (1 - cos(pi * x));
    elseif distTraveled <= rampCounts
        x         = max(0.0, min(1.0, distTraveled / rampCounts));
        targetRPM = MIN_RPM + (peakRPM - MIN_RPM) * 0.5 * (1 - cos(pi * x));
    else
        targetRPM = peakRPM;
    end
    currentRPM = max(MIN_RPM, min(speedRPM, targetRPM));

    % -------------------------------------------------------------------------
    % 7. DDS PULSE ACCUMULATOR
    % -------------------------------------------------------------------------
    if startNext && absError > STOP_COUNTS
        pulseAccum = pulseAccum + currentRPM * C2R * Ts;
        if pulseAccum >= 1.0
            pul          = 1;
            pulseAccum   = pulseAccum - 1.0;
            distTraveled = distTraveled + 1;
        end
        next = false;
    else
        next       = (absError <= STOP_COUNTS);
        pulseAccum = 0;
    end

    % -------------------------------------------------------------------------
    % 8. LIMIT SWITCH SAFETY (modes 0 and 1 only)
    % -------------------------------------------------------------------------
    if homedFlag && currentCount > LIMIT_BUFFER
        homedFlag = false;
    end
    if rst == 1 && ~homedFlag && dir == 0
        limit = true;
        pul   = 0;
    end
    if currentCount > maxCount
        limit = true;
        pul   = 0;
    end

    % -------------------------------------------------------------------------
    % 8.5 MODE-0 PULSE SUPPRESSION
    %     In position mode, CoordMove owns all pulse/dir generation.
    %     Force this block's own pul/dir to 0 so it can't leak a second
    %     pulse stream to the driver. Encoder counting + limit safety above
    %     still run normally every tick.
    % -------------------------------------------------------------------------
    if mode == 0
        pul = 0;
    end


    % -------------------------------------------------------------------------
    % 9. OUTPUTS
    % -------------------------------------------------------------------------
    count        = currentCount;
    displaySpeed = smoothedSpeed;
    homed        = homedFlag;
    lastClkState = clk;

end

== matlab function AR4FullPositionControl/Subsystem/J5/MATLAB Function1 ==
  data: startNext input; clk input; count output; dt input; rst input; displaySpeed output; dir output; pul output; next output; speedRPM input; positionAngle input; currCount input; accelRPMperSec input; limit output; mode input; homed output
function [count, displaySpeed, dir, pul, next, limit, homed] = J5(startNext, clk, dt, rst, speedRPM, positionAngle, currCount, accelRPMperSec, mode)
% J5 - Joint 5 position/speed controller with S-curve acceleration + HOMING
%
%   >>> J5: span=208.5 deg (108.5-...-100)  maxCount=5800  HOME_TARGET=90
%   >>> Backlash compensation added (~7 deg measured play)

    persistent currentCount lastClkState lastCount spTimer smoothedSpeed ...
               currentRPM distTraveled totalMoveFrozen lastTarget pulseAccum ...
               homedFlag lastMode lastRawCmd backlashSign;

    % -------------------------------------------------------------------------
    % CONSTANTS  -  per-joint values
    % -------------------------------------------------------------------------
    Ts           = 3e-5;
    PPR          = 1000;
    CPR          = PPR * 4;
    maxCount     = 5800;           % <<< J5
    LIMIT_BUFFER = 50;
    TUNE_C2R     = 1.6;            % <<< J5

    TOTAL_DEG      = 208.5;          % <<< J5 span: 108.5-(-100)
    COUNTS_PER_REV = maxCount / TOTAL_DEG * 360;
    GEAR_RATIO     = COUNTS_PER_REV / CPR;
    C2R            = (GEAR_RATIO * CPR) / 60 * TUNE_C2R;

    speedUpdateInterval = 0.2;
    ALPHA               = 0.3;
    MIN_RPM             = 0.5;
    STOP_COUNTS         = 1;

    HOME_RPM    = 5;               % <<< tune: homing speed (RPM)
    HOME_TARGET = 90;              % <<< J5 home angle (deg)

    % Single-limit angle->count mapping (anchored at switch)
    J_MIN_DEG    = -100;           % <<< J5
    J_MAX_DEG    =  108.5;           % <<< J5
    SWITCH_DEG   = -100;           % <<< J5 switch at -100 deg = count 0
    countsPerDeg = maxCount / TOTAL_DEG;

    % -------------------------------------------------------------------------
    % INITIALISATION (first call only)
    % -------------------------------------------------------------------------
    if isempty(currentCount)
        currentCount    = currCount;
        lastCount       = currCount;
        lastClkState    = clk;
        spTimer         = 0;
        smoothedSpeed   = 0;
        currentRPM      = MIN_RPM;
        distTraveled    = 0;
        totalMoveFrozen = 0;
        lastTarget      = -1;
        pulseAccum      = 0;
        homedFlag       = false;
        lastMode        = 0;
        lastRawCmd      = -999;    % force first target to register as "new"
        backlashSign    = 0;
    end

    limit = false;
    homed = homedFlag;
    dir   = 0;
    pul   = 0;
    next  = false;

    % -------------------------------------------------------------------------
    % 1. ENCODER COUNTING
    % -------------------------------------------------------------------------
    if clk ~= lastClkState && clk == 1
        if dt ~= clk
            currentCount = currentCount + 1;
        else
            currentCount = currentCount - 1;
        end
    end

    % Reset S-curve state on any mode change (once, on the transition)
    if mode ~= lastMode
        distTraveled    = 0;
        totalMoveFrozen = 0;
        pulseAccum      = 0;
        lastTarget      = -1;
        currentRPM      = MIN_RPM;
        spTimer         = 0;
        smoothedSpeed   = 0;
    end
    lastMode = mode;

    % =========================================================================
    % MODE 2: HOMING
    % =========================================================================
    if mode == 2
        if rst == 1
            currentCount = 0;
            homedFlag    = true;
        end
        homed = homedFlag;          % limit NOT asserted during homing

        if homedFlag
            currentCount = 0;
            pul          = 0;
            next         = true;
        elseif startNext
            dir        = 0;         % toward switch = decreasing count
            pulseAccum = pulseAccum + HOME_RPM * C2R * Ts;
            if pulseAccum >= 1.0
                pul        = 1;
                pulseAccum = pulseAccum - 1.0;
            end
        end

        count        = currentCount;
        displaySpeed = HOME_RPM;
        lastClkState = clk;
        return;
    end
    % =========================================================================

    % -------------------------------------------------------------------------
    % 2. SPEED DISPLAY
    % -------------------------------------------------------------------------
    spTimer = spTimer + Ts;
    if spTimer >= speedUpdateInterval
        smoothedSpeed = ALPHA * currentRPM + (1 - ALPHA) * smoothedSpeed;
        spTimer       = 0;
    end

    % -------------------------------------------------------------------------
    % 3. TARGET FROM ANGLE
    % -------------------------------------------------------------------------
    if mode == 1
        cmdAngle = HOME_TARGET;
    else
        cmdAngle = positionAngle;
    end

    % ---------------------------------------------------------------------
    % BACKLASH COMPENSATION (J5: ~7 deg measured play, stable)
    % Latch compensation direction ONCE when a NEW target arrives (based on
    % travel direction from current physical position), then HOLD it for the
    % whole move. Holding (not recomputing every cycle) is what makes it
    % work -- otherwise arrival at the target erases the offset.
    % ---------------------------------------------------------------------
    BACKLASH_DEG = 7.0;             % <<< measured J5 backlash (tune)
    halfBacklash = BACKLASH_DEG / 2;

    rawTarget = cmdAngle;           % uncompensated commanded angle

    if abs(rawTarget - lastRawCmd) > 0.5     % a NEW target was commanded
        currentAngle = SWITCH_DEG + (currentCount / countsPerDeg);
        if rawTarget > currentAngle
            backlashSign = 1;       % must move + -> shift target +
        elseif rawTarget < currentAngle
            backlashSign = -1;      % must move - -> shift target -
        else
            backlashSign = 0;
        end
        lastRawCmd = rawTarget;
    end
    % backlashSign persists (held) across calls for the whole move

    cmdAngle = rawTarget + backlashSign * halfBacklash;

    % Clamp to physical range, then map (single-limit, anchored at switch)
    if cmdAngle < J_MIN_DEG, cmdAngle = J_MIN_DEG; end
    if cmdAngle > J_MAX_DEG, cmdAngle = J_MAX_DEG; end
    targetCount = round(abs(SWITCH_DEG - cmdAngle) * countsPerDeg);
    targetCount = max(LIMIT_BUFFER, min(maxCount - LIMIT_BUFFER, targetCount));

    % -------------------------------------------------------------------------
    % 4. DIRECTION
    % -------------------------------------------------------------------------
    countError = targetCount - currentCount;
    absError   = abs(countError);
    if countError >= 0
        dir = 1;
    else
        dir = 0;
    end

    % -------------------------------------------------------------------------
    % 5. FREEZE totalMove ON NEW TARGET
    % -------------------------------------------------------------------------
    if targetCount ~= lastTarget
        totalMoveFrozen = absError;
        distTraveled    = 0;
        pulseAccum      = 0;
        lastTarget      = targetCount;
    end

    % -------------------------------------------------------------------------
    % 6. S-CURVE SPEED PROFILE
    % -------------------------------------------------------------------------
    accel = max(accelRPMperSec, 0.1);
    fullRampCounts = 0.5 * (MIN_RPM + speedRPM) * C2R * (speedRPM - MIN_RPM) / accel;

    if totalMoveFrozen > 0 && 2 * fullRampCounts >= totalMoveFrozen
        peakRPM    = sqrt(max(MIN_RPM^2 + totalMoveFrozen * accel / C2R, MIN_RPM^2));
        peakRPM    = max(MIN_RPM, min(speedRPM, peakRPM));
        rampCounts = 0.5 * (MIN_RPM + peakRPM) * C2R * (peakRPM - MIN_RPM) / accel;
        rampCounts = max(1, rampCounts);
    else
        peakRPM    = speedRPM;
        rampCounts = max(1, fullRampCounts);
    end

    if totalMoveFrozen <= 0
        targetRPM = MIN_RPM;
    elseif absError <= rampCounts
        x         = max(0.0, min(1.0, absError / rampCounts));
        targetRPM = MIN_RPM + (peakRPM - MIN_RPM) * 0.5 * (1 - cos(pi * x));
    elseif distTraveled <= rampCounts
        x         = max(0.0, min(1.0, distTraveled / rampCounts));
        targetRPM = MIN_RPM + (peakRPM - MIN_RPM) * 0.5 * (1 - cos(pi * x));
    else
        targetRPM = peakRPM;
    end
    currentRPM = max(MIN_RPM, min(speedRPM, targetRPM));

    % -------------------------------------------------------------------------
    % 7. DDS PULSE ACCUMULATOR
    % -------------------------------------------------------------------------
    if startNext && absError > STOP_COUNTS
        pulseAccum = pulseAccum + currentRPM * C2R * Ts;
        if pulseAccum >= 1.0
            pul          = 1;
            pulseAccum   = pulseAccum - 1.0;
            distTraveled = distTraveled + 1;
        end
        next = false;
    else
        next       = (absError <= STOP_COUNTS);
        pulseAccum = 0;
    end

    % -------------------------------------------------------------------------
    % 8. LIMIT SWITCH SAFETY (modes 0 and 1 only)
    % -------------------------------------------------------------------------
    if homedFlag && currentCount > LIMIT_BUFFER
        homedFlag = false;
    end
    if rst == 1 && ~homedFlag && dir == 0
        limit = true;
        pul   = 0;
    end
    if currentCount > maxCount
        limit = true;
        pul   = 0;
    end

    % -------------------------------------------------------------------------
    % 8.5 MODE-0 PULSE SUPPRESSION
    %     In position mode, CoordMove owns all pulse/dir generation.
    %     Force this block's own pul/dir to 0 so it can't leak a second
    %     pulse stream to the driver. Encoder counting + limit safety above
    %     still run normally every tick.
    % -------------------------------------------------------------------------
    if mode == 0
        pul = 0;
    end


    % -------------------------------------------------------------------------
    % 9. OUTPUTS
    % -------------------------------------------------------------------------
    count        = currentCount;
    displaySpeed = smoothedSpeed;
    homed        = homedFlag;
    lastClkState = clk;

end
